simulink model "sesion2_act2"  (R2021a)
settings: Solver=ode1  StartTime=0.0  StopTime=30.0  FixedStep=0.001  RelTol=1e-3
libraries: cstblocks x3
settings Model: Creator=zeta  LastModifiedBy=zeta

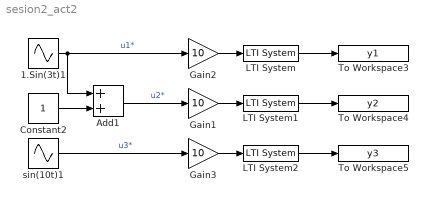
== system sesion2_act2 ==
  1.Sin(3t)1 : Sin  Frequency=3  SampleTime=0
  Add1 : Sum
  Constant2 : Constant
  Gain1 : Gain  Gain=10
  Gain2 : Gain  Gain=10
  Gain3 : Gain  Gain=10
  LTI System : cstblocks/LTI System  sys=sys  IC=[]
  LTI System1 : cstblocks/LTI System  sys=sys  IC=[]
  LTI System2 : cstblocks/LTI System  sys=sys  IC=[]
  To Workspace3 : ToWorkspace  VariableName=y1  SampleTime=-1
  To Workspace4 : ToWorkspace  VariableName=y2  SampleTime=-1
  To Workspace5 : ToWorkspace  VariableName=y3  SampleTime=-1
  sin(10t)1 : Sin  Frequency=10  SampleTime=0
  wires:
  Constant2/1 -> Add1/2
  Add1/1 -> Gain1/1  "u2*"
  sin(10t)1/1 -> Gain3/1  "u3*"
  1.Sin(3t)1/1 -> Gain2/1, Add1/1  "u1*"
  Gain1/1 -> LTI System1/1
  Gain2/1 -> LTI System/1
  Gain3/1 -> LTI System2/1
  LTI System/1 -> To Workspace3/1
  LTI System1/1 -> To Workspace4/1
  LTI System2/1 -> To Workspace5/1
